simulink model "untitled"  (R2019a)
settings: Solver=VariableStepAuto  StartTime=0.0  StopTime=10.0  RelTol=1e-3
settings Model: Creator=ASUS_PEPE  LastModifiedBy=ASUS_PEPE
settings SolverCC: AlgebraicLoopSolver=LineSearch

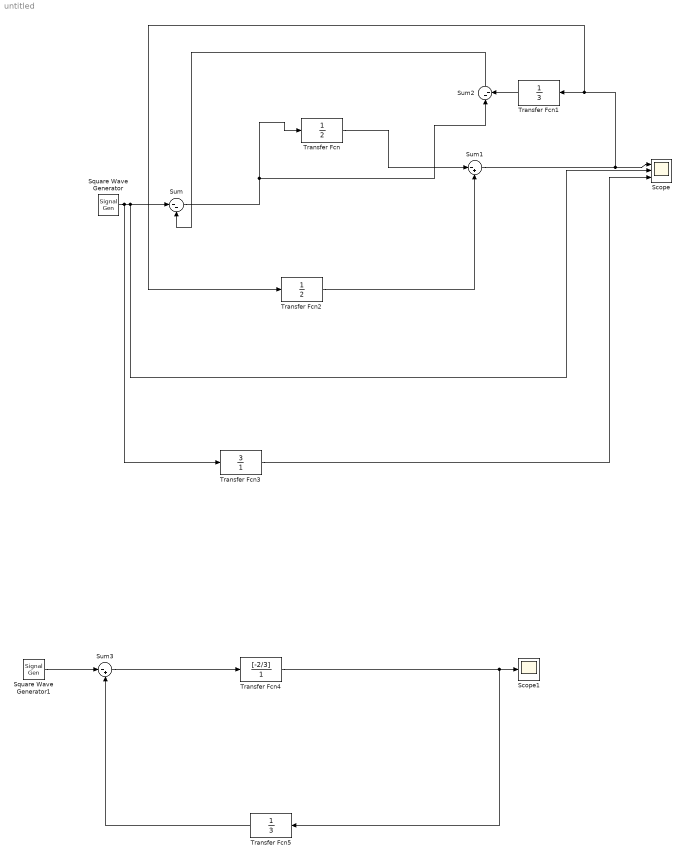
== system untitled ==
  Scope : Scope  NumInputPorts=3
  Scope1 : Scope
  Square Wave Generator : SignalGenerator  WaveForm=square  Units=rad/sec
  Square Wave Generator1 : SignalGenerator  WaveForm=square  Units=rad/sec
  Sum : Sum  Inputs=|--
  Sum1 : Sum  Inputs=|-+
  Sum2 : Sum  Inputs=|--
  Sum3 : Sum  Inputs=|-+
  Transfer Fcn : TransferFcn  Denominator=[0 2]
  Transfer Fcn1 : TransferFcn  Denominator=[0 3]
  Transfer Fcn2 : TransferFcn  Denominator=[0 2]
  Transfer Fcn3 : TransferFcn  Numerator=[3]  Denominator=[0 1]
  Transfer Fcn4 : TransferFcn  Numerator=[-2/3]  Denominator=[0 1]
  Transfer Fcn5 : TransferFcn  Denominator=[0 3]
  wires:
  Transfer Fcn/1 -> Sum1/1
  Sum2/1 -> Sum/2
  Sum/1 -> Transfer Fcn/1, Sum2/1
  Transfer Fcn1/1 -> Sum2/2
  Transfer Fcn2/1 -> Sum1/2
  Sum1/1 -> Transfer Fcn1/1, Transfer Fcn2/1, Scope/1
  Square Wave Generator/1 -> Transfer Fcn3/1, Scope/2, Sum/1
  Transfer Fcn3/1 -> Scope/3
  Square Wave Generator1/1 -> Sum3/1
  Transfer Fcn4/1 -> Transfer Fcn5/1, Scope1/1
  Transfer Fcn5/1 -> Sum3/2
  Sum3/1 -> Transfer Fcn4/1
